simulink model "controllo_disco_rigido_closedloop"  (R2019b)
settings: Solver=VariableStepAuto  StartTime=0.0  StopTime=10.0  RelTol=1e-3
values from neighbouring files (symbols this model uses):
  b = 0.002    [controllo_disco_rigido.m]    (also in controllo_disco_rigido_baseWS.mat; controllo_disco_rigido_script.m; init_controllo_disco_rigido.m)
  J = 0.001    [controllo_disco_rigido.m]    (also in controllo_disco_rigido_baseWS.mat; controllo_disco_rigido_script.m; init_controllo_disco_rigido.m)
  y0 = 300    [controllo_disco_rigido.m]    (also in controllo_disco_rigido_script.m)
settings Model: Creator=Utente  LastModifiedBy=Utente

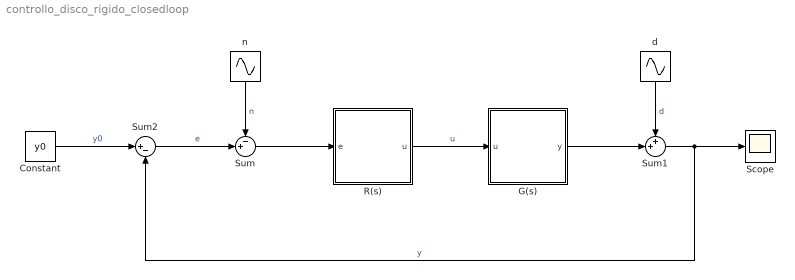
== system controllo_disco_rigido_closedloop ==
  Constant : Constant  Value=y0
  G(s) : Subsystem
  R(s) : Subsystem
  Scope : Scope
  Sum : Sum  Inputs=-+|
  Sum1 : Sum  Inputs=++|
  Sum2 : Sum  Inputs=|+-
  d : Sin  Frequency=[0.5, 5]  SampleTime=0
  n : Sin  Frequency=[50, 500]  SampleTime=0
  wires:
  R(s)/1(u) -> G(s)/1(u)  "u"
  Sum/1 -> R(s)/1(e)
  G(s)/1(y) -> Sum1/2
  Sum1/1 -> Sum2/2, Scope/1  "y"
  Sum2/1 -> Sum/2  "e"
  Constant/1 -> Sum2/1  "y0"
  d/1 -> Sum1/1  "d"
  n/1 -> Sum/1  "n"

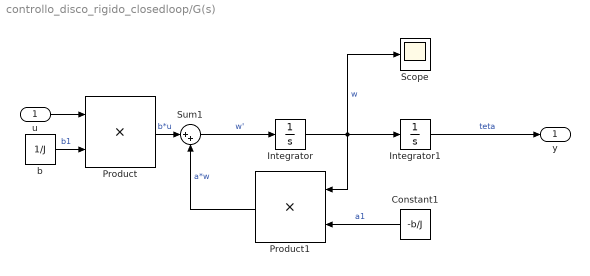
== system controllo_disco_rigido_closedloop/G(s) ==
  u : Inport
  Constant1 : Constant  Value=-b/J
  Integrator : Integrator
  Integrator1 : Integrator
  Product : Product
  Product1 : Product
  Scope : Scope
  Sum1 : Sum  Inputs=|++
  b : Constant  Value=1/J
  y : Outport
  wires:
  Integrator/1 -> Scope/1, Integrator1/1, Product1/1  "w"
  b/1 -> Product/2  "b1"
  u/1 -> Product/1
  Product/1 -> Sum1/1  "b*u"
  Constant1/1 -> Product1/2  "a1"
  Integrator1/1 -> y/1  "teta"
  Sum1/1 -> Integrator/1  "w'"
  Product1/1 -> Sum1/2  "a*w"

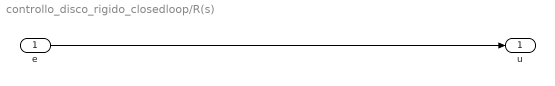
== system controllo_disco_rigido_closedloop/R(s) ==
  e : Inport
  u : Outport
  wires:
  e/1 -> u/1
